simulink model "task3_dcm"  (R2017a)
settings: Solver=VariableStepAuto  StartTime=0.0  StopTime=0.5  MaxStep=1e-4  RelTol=1e-3
undefined symbols (not defined in the file): ki, kp, Ra, Vbase
settings Model: Creator=Oskar  LastModifiedBy=Oskar

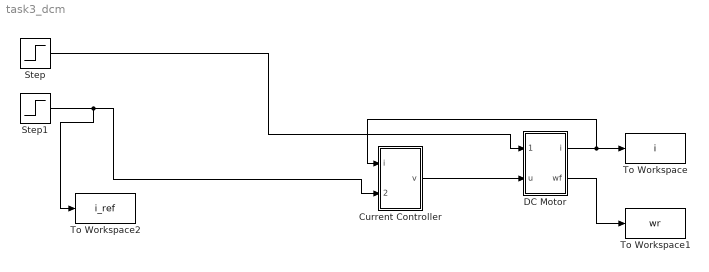
== system task3_dcm ==
  Current Controller : Subsystem
  "DC Motor " : Subsystem  mask{R=0.5, L=2.5/1000, psi=0.35, J=1e-3}
      mask prompts: R "R (ohm)"; L "L (H)"; psi "psi (Vs)"; J "J (kgm^2)"
      mask TypeOptions R: <empty>
  Step : Step  Time=0.3  After=7  SampleTime=0
  Step1 : Step  Time=0.1  After=20  SampleTime=0
  To Workspace : ToWorkspace  VariableName=i  SaveFormat=Timeseries  SampleTime=-1
  To Workspace1 : ToWorkspace  VariableName=wr  SaveFormat=Timeseries  SampleTime=-1
  To Workspace2 : ToWorkspace  VariableName=i_ref  SaveFormat=Timeseries  SampleTime=-1
  wires:
  "DC Motor "/1("i ") -> Current Controller/1(i), To Workspace/1
  "DC Motor "/2("wf ") -> To Workspace1/1
  Current Controller/1(v) -> "DC Motor "/2(u)
  Step/1 -> "DC Motor "/1("taul ")
  Step1/1 -> To Workspace2/1, Current Controller/2("i_ref ")

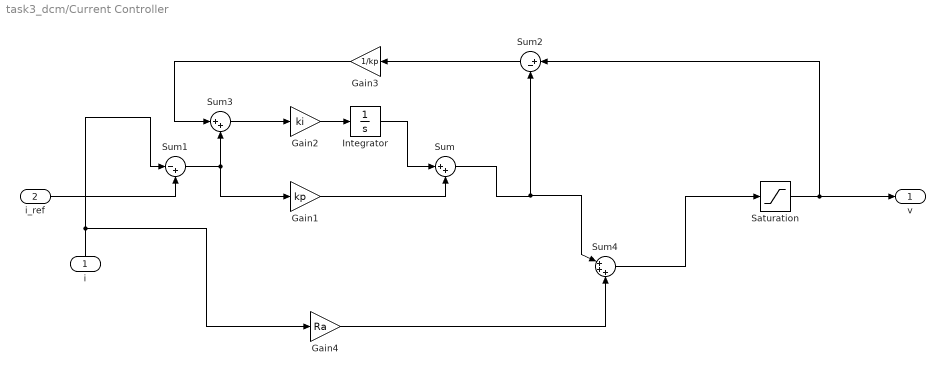
== system task3_dcm/Current Controller ==
  i : Inport
  "i_ref " : Inport  Port=2
  Gain1 : Gain  Gain=kp
  Gain2 : Gain  Gain=ki
  Gain3 : Gain  Gain=1/kp
  Gain4 : Gain  Gain=Ra
  Integrator : Integrator
  Saturation : Saturate  UpperLimit=Vbase  LowerLimit=-Vbase
  Sum : Sum  Inputs=|++
  Sum1 : Sum  Inputs=|-+
  Sum2 : Sum  Inputs=|+-
  Sum3 : Sum  Inputs=|++
  Sum4 : Sum  Inputs=|+++
  v : Outport
  wires:
  "i_ref "/1 -> Sum1/2
  Gain2/1 -> Integrator/1
  Integrator/1 -> Sum/1
  Gain1/1 -> Sum/2
  Saturation/1 -> v/1, Sum2/1
  Sum2/1 -> Gain3/1
  Sum/1 -> Sum4/1, Sum2/2
  Sum1/1 -> Gain1/1, Sum3/2
  Gain3/1 -> Sum3/1
  i/1 -> Gain4/1, Sum1/1
  Sum3/1 -> Gain2/1
  Gain4/1 -> Sum4/3
  Sum4/1 -> Saturation/1

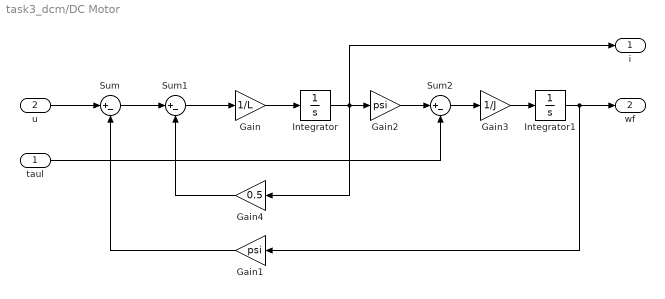
== system task3_dcm/DC Motor  ==
  "taul " : Inport
  u : Inport  Port=2
  Gain : Gain  Gain=1/L
  Gain1 : Gain  Gain=psi
  Gain2 : Gain  Gain=psi
  Gain3 : Gain  Gain=1/J
  Gain4 : Gain  Gain=0.5
  Integrator : Integrator
  Integrator1 : Integrator
  Sum : Sum  Inputs=|+-
  Sum1 : Sum  Inputs=|+-
  Sum2 : Sum  Inputs=|+-
  "i " : Outport
  "wf " : Outport  Port=2
  wires:
  Integrator1/1 -> "wf "/1, Gain1/1
  Sum2/1 -> Gain3/1
  Gain3/1 -> Integrator1/1
  Gain2/1 -> Sum2/1
  Gain4/1 -> Sum1/2
  Sum/1 -> Sum1/1
  u/1 -> Sum/1
  Sum1/1 -> Gain/1
  Gain/1 -> Integrator/1
  "taul "/1 -> Sum2/2
  Integrator/1 -> "i "/1, Gain4/1, Gain2/1
  Gain1/1 -> Sum/2
